simulink model "TST_Tra_GearInfo"  (R2016b)
settings: Solver=FixedStepDiscrete  StartTime=0.0  StopTime=simTime  FixedStep=sampleTime  RelTol=1e-3
values from neighbouring files (symbols this model uses):
  testCase = 1    [initTST_Tra_GearInfo_001.m]
libraries: simulink x11, UnitTest_Lib x9
settings Model: Creator=zhengjinyan  LastModifiedBy=zhengjinyan
settings DebuggingCC: SignalRangeChecking=error

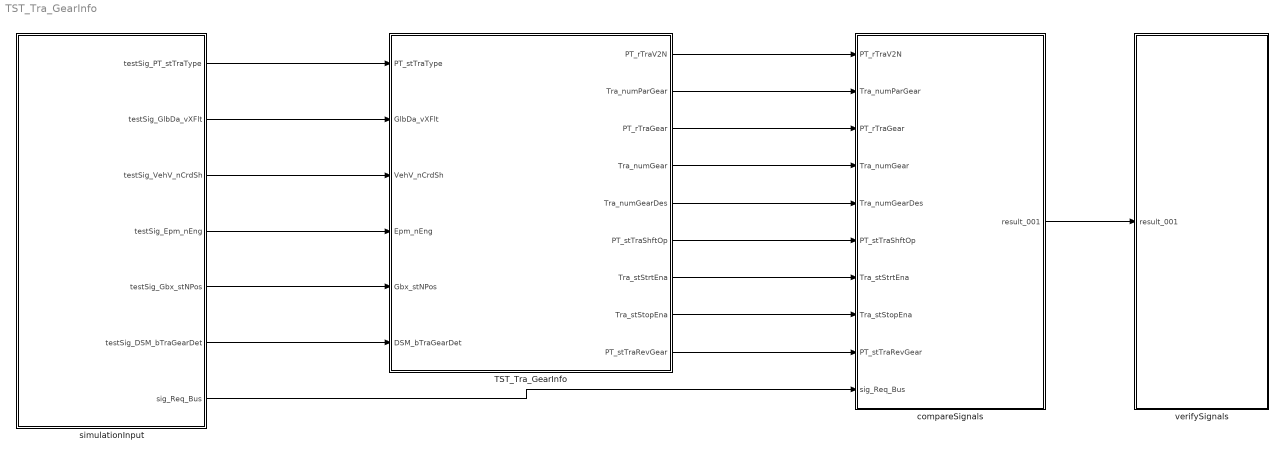
== system TST_Tra_GearInfo ==
  TST_Tra_GearInfo : Subsystem
  compareSignals : Subsystem
  simulationInput : Subsystem
  verifySignals : Subsystem
  wires:
  simulationInput/1(testSig_PT_stTraType) -> TST_Tra_GearInfo/1(PT_stTraType)
  simulationInput/2(testSig_GlbDa_vXFlt) -> TST_Tra_GearInfo/2(GlbDa_vXFlt)
  simulationInput/3(testSig_VehV_nCrdSh) -> TST_Tra_GearInfo/3(VehV_nCrdSh)
  simulationInput/4(testSig_Epm_nEng) -> TST_Tra_GearInfo/4(Epm_nEng)
  simulationInput/5(testSig_Gbx_stNPos) -> TST_Tra_GearInfo/5(Gbx_stNPos)
  simulationInput/6(testSig_DSM_bTraGearDet) -> TST_Tra_GearInfo/6(DSM_bTraGearDet)
  TST_Tra_GearInfo/1(PT_rTraV2N) -> compareSignals/1(PT_rTraV2N)
  TST_Tra_GearInfo/2(Tra_numParGear) -> compareSignals/2(Tra_numParGear)
  TST_Tra_GearInfo/3(PT_rTraGear) -> compareSignals/3(PT_rTraGear)
  TST_Tra_GearInfo/4(Tra_numGear) -> compareSignals/4(Tra_numGear)
  TST_Tra_GearInfo/5(Tra_numGearDes) -> compareSignals/5(Tra_numGearDes)
  TST_Tra_GearInfo/6(PT_stTraShftOp) -> compareSignals/6(PT_stTraShftOp)
  TST_Tra_GearInfo/7(Tra_stStrtEna) -> compareSignals/7(Tra_stStrtEna)
  TST_Tra_GearInfo/8(Tra_stStopEna) -> compareSignals/8(Tra_stStopEna)
  TST_Tra_GearInfo/9(PT_stTraRevGear) -> compareSignals/9(PT_stTraRevGear)
  simulationInput/7(sig_Req_Bus) -> compareSignals/10(sig_Req_Bus)
  compareSignals/1(result_001) -> verifySignals/1(result_001)

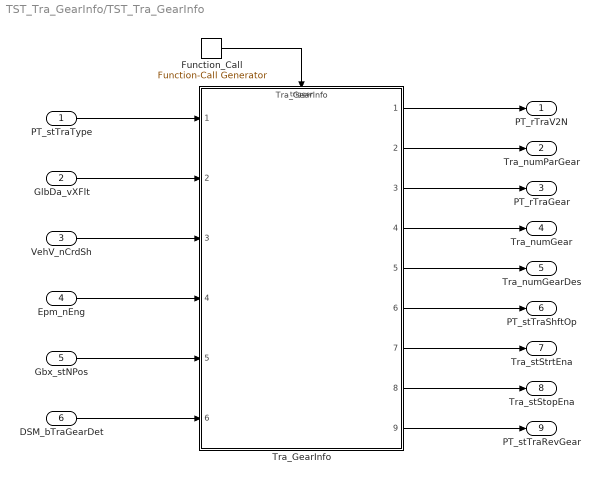
== system TST_Tra_GearInfo/TST_Tra_GearInfo ==
  PT_stTraType : Inport
  GlbDa_vXFlt : Inport  Port=2
  VehV_nCrdSh : Inport  Port=3
  Epm_nEng : Inport  Port=4
  Gbx_stNPos : Inport  Port=5
  DSM_bTraGearDet : Inport  Port=6
  Function_Call : simulink/Ports & Subsystems/Function-Call Generator  sample_time=sampleTime  numberOfIterations=1
  Tra_GearInfo : ModelReference  ModelNameDialog=Tra_GearInfo  SimulationMode=Normal  ModelReferenceVersion=1.62  TriggerPortName=function  TriggerPortTriggerType=function-call  TriggerPortStatesWhenEnabling=held
  PT_rTraV2N : Outport
  Tra_numParGear : Outport  Port=2
  PT_rTraGear : Outport  Port=3
  Tra_numGear : Outport  Port=4
  Tra_numGearDes : Outport  Port=5
  PT_stTraShftOp : Outport  Port=6
  Tra_stStrtEna : Outport  Port=7
  Tra_stStopEna : Outport  Port=8
  PT_stTraRevGear : Outport  Port=9
  wires:
  Function_Call/1 -> Tra_GearInfo/Trigger
  PT_stTraType/1 -> Tra_GearInfo/1
  GlbDa_vXFlt/1 -> Tra_GearInfo/2
  VehV_nCrdSh/1 -> Tra_GearInfo/3
  Epm_nEng/1 -> Tra_GearInfo/4
  Gbx_stNPos/1 -> Tra_GearInfo/5
  DSM_bTraGearDet/1 -> Tra_GearInfo/6
  Tra_GearInfo/1 -> PT_rTraV2N/1
  Tra_GearInfo/2 -> Tra_numParGear/1
  Tra_GearInfo/3 -> PT_rTraGear/1
  Tra_GearInfo/4 -> Tra_numGear/1
  Tra_GearInfo/5 -> Tra_numGearDes/1
  Tra_GearInfo/6 -> PT_stTraShftOp/1
  Tra_GearInfo/7 -> Tra_stStrtEna/1
  Tra_GearInfo/8 -> Tra_stStopEna/1
  Tra_GearInfo/9 -> PT_stTraRevGear/1

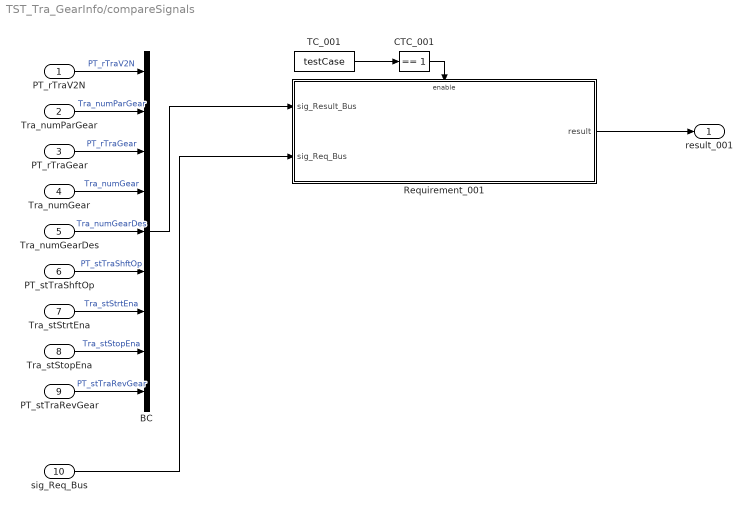
== system TST_Tra_GearInfo/compareSignals ==
  PT_rTraV2N : Inport
  Tra_numParGear : Inport  Port=2
  PT_rTraGear : Inport  Port=3
  Tra_numGear : Inport  Port=4
  Tra_numGearDes : Inport  Port=5
  PT_stTraShftOp : Inport  Port=6
  Tra_stStrtEna : Inport  Port=7
  Tra_stStopEna : Inport  Port=8
  PT_stTraRevGear : Inport  Port=9
  sig_Req_Bus : Inport  Port=10
  BC : BusCreator  Inputs=9
  CTC_001 : simulink/Logic and Bit Operations/Compare To Constant  relop===  const=1  OutDataTypeStr=boolean
  Requirement_001 : Subsystem
  TC_001 : Constant  Value=testCase
  result_001 : Outport
  wires:
  PT_rTraV2N/1 -> BC/1  "PT_rTraV2N"
  Tra_numParGear/1 -> BC/2  "Tra_numParGear"
  PT_rTraGear/1 -> BC/3  "PT_rTraGear"
  Tra_numGear/1 -> BC/4  "Tra_numGear"
  Tra_numGearDes/1 -> BC/5  "Tra_numGearDes"
  PT_stTraShftOp/1 -> BC/6  "PT_stTraShftOp"
  Tra_stStrtEna/1 -> BC/7  "Tra_stStrtEna"
  Tra_stStopEna/1 -> BC/8  "Tra_stStopEna"
  PT_stTraRevGear/1 -> BC/9  "PT_stTraRevGear"
  TC_001/1 -> CTC_001/1
  CTC_001/1 -> Requirement_001/Enable
  sig_Req_Bus/1 -> Requirement_001/2(sig_Req_Bus)
  BC/1 -> Requirement_001/1(sig_Result_Bus)
  Requirement_001/1(result) -> result_001/1

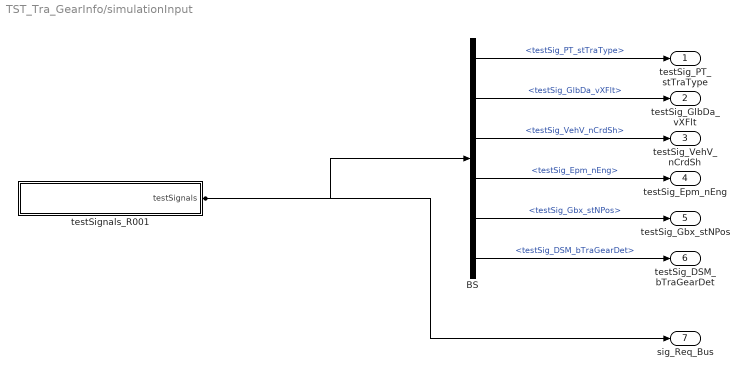
== system TST_Tra_GearInfo/simulationInput ==
  BS : BusSelector  OutputSignals=testSig_PT_stTraType,testSig_GlbDa_vXFlt,testSig_VehV_nCrdSh,testSig_Epm_nEng,testSig_Gbx_stNPos,testSig_DSM_bTraGearDet
  testSignals_R001 : Subsystem
  testSig_PT_stTraType : Outport
  testSig_GlbDa_vXFlt : Outport  Port=2
  testSig_VehV_nCrdSh : Outport  Port=3
  testSig_Epm_nEng : Outport  Port=4
  testSig_Gbx_stNPos : Outport  Port=5
  testSig_DSM_bTraGearDet : Outport  Port=6
  sig_Req_Bus : Outport  Port=7
  wires:
  BS/1 -> testSig_PT_stTraType/1  "<testSig_PT_stTraType>"
  BS/2 -> testSig_GlbDa_vXFlt/1  "<testSig_GlbDa_vXFlt>"
  BS/3 -> testSig_VehV_nCrdSh/1  "<testSig_VehV_nCrdSh>"
  BS/4 -> testSig_Epm_nEng/1  "<testSig_Epm_nEng>"
  BS/5 -> testSig_Gbx_stNPos/1  "<testSig_Gbx_stNPos>"
  BS/6 -> testSig_DSM_bTraGearDet/1  "<testSig_DSM_bTraGearDet>"
  testSignals_R001/1(testSignals) -> BS/1, sig_Req_Bus/1

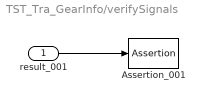
== system TST_Tra_GearInfo/verifySignals ==
  result_001 : Inport
  Assertion_001 : Assertion  Enabled=off
  wires:
  result_001/1 -> Assertion_001/1

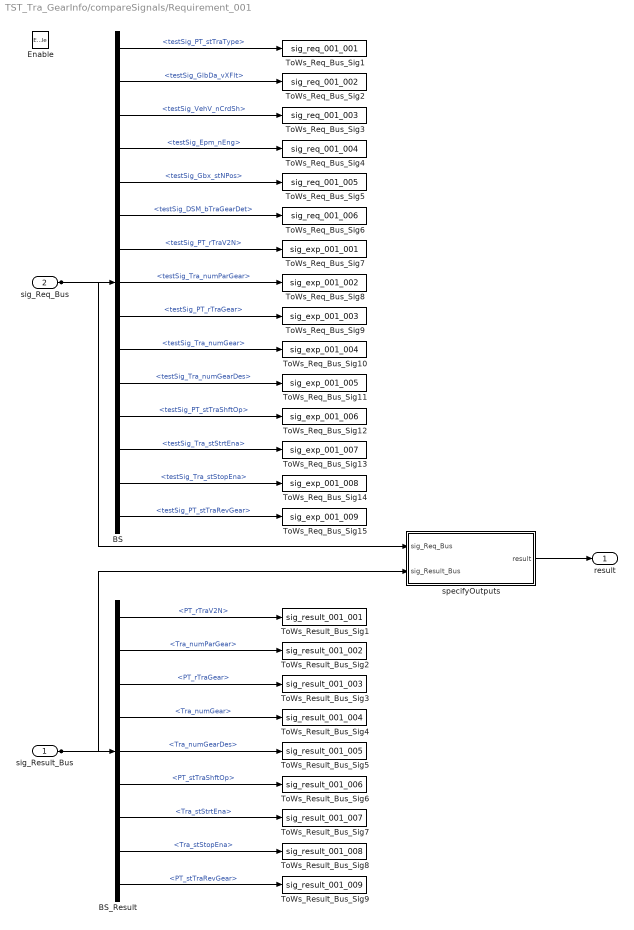
== system TST_Tra_GearInfo/compareSignals/Requirement_001 ==
  sig_Result_Bus : Inport
  sig_Req_Bus : Inport  Port=2
  Enable : EnablePort
  BS : BusSelector  OutputSignals=testSig_PT_stTraType,testSig_GlbDa_vXFlt,testSig_VehV_nCrdSh,testSig_Epm_nEng,testSig_Gbx_stNPos,testSig_DSM_bTraGearDet,testSig_PT_rTraV2N,testSig_Tra_numParGear,testSig_PT_rTraGear,testSig_Tra_numGear,testSig_Tra_numGearDes,testSig_PT_stTraShftOp,testSig_Tra_stStrtEna,testSig_Tra_stStopEna,testSig_PT_stTraRevGear
  BS_Result : BusSelector  OutputSignals=PT_rTraV2N,Tra_numParGear,PT_rTraGear,Tra_numGear,Tra_numGearDes,PT_stTraShftOp,Tra_stStrtEna,Tra_stStopEna,PT_stTraRevGear
  ToWs_Req_Bus_Sig1 : ToWorkspace  VariableName=sig_req_001_001  SaveFormat=Structure With Time
  ToWs_Req_Bus_Sig10 : ToWorkspace  VariableName=sig_exp_001_004  SaveFormat=Structure With Time
  ToWs_Req_Bus_Sig11 : ToWorkspace  VariableName=sig_exp_001_005  SaveFormat=Structure With Time
  ToWs_Req_Bus_Sig12 : ToWorkspace  VariableName=sig_exp_001_006  SaveFormat=Structure With Time
  ToWs_Req_Bus_Sig13 : ToWorkspace  VariableName=sig_exp_001_007  SaveFormat=Structure With Time
  ToWs_Req_Bus_Sig14 : ToWorkspace  VariableName=sig_exp_001_008  SaveFormat=Structure With Time
  ToWs_Req_Bus_Sig15 : ToWorkspace  VariableName=sig_exp_001_009  SaveFormat=Structure With Time
  ToWs_Req_Bus_Sig2 : ToWorkspace  VariableName=sig_req_001_002  SaveFormat=Structure With Time
  ToWs_Req_Bus_Sig3 : ToWorkspace  VariableName=sig_req_001_003  SaveFormat=Structure With Time
  ToWs_Req_Bus_Sig4 : ToWorkspace  VariableName=sig_req_001_004  SaveFormat=Structure With Time
  ToWs_Req_Bus_Sig5 : ToWorkspace  VariableName=sig_req_001_005  SaveFormat=Structure With Time
  ToWs_Req_Bus_Sig6 : ToWorkspace  VariableName=sig_req_001_006  SaveFormat=Structure With Time
  ToWs_Req_Bus_Sig7 : ToWorkspace  VariableName=sig_exp_001_001  SaveFormat=Structure With Time
  ToWs_Req_Bus_Sig8 : ToWorkspace  VariableName=sig_exp_001_002  SaveFormat=Structure With Time
  ToWs_Req_Bus_Sig9 : ToWorkspace  VariableName=sig_exp_001_003  SaveFormat=Structure With Time
  ToWs_Result_Bus_Sig1 : ToWorkspace  VariableName=sig_result_001_001  SaveFormat=Structure With Time
  ToWs_Result_Bus_Sig2 : ToWorkspace  VariableName=sig_result_001_002  SaveFormat=Structure With Time
  ToWs_Result_Bus_Sig3 : ToWorkspace  VariableName=sig_result_001_003  SaveFormat=Structure With Time
  ToWs_Result_Bus_Sig4 : ToWorkspace  VariableName=sig_result_001_004  SaveFormat=Structure With Time
  ToWs_Result_Bus_Sig5 : ToWorkspace  VariableName=sig_result_001_005  SaveFormat=Structure With Time
  ToWs_Result_Bus_Sig6 : ToWorkspace  VariableName=sig_result_001_006  SaveFormat=Structure With Time
  ToWs_Result_Bus_Sig7 : ToWorkspace  VariableName=sig_result_001_007  SaveFormat=Structure With Time
  ToWs_Result_Bus_Sig8 : ToWorkspace  VariableName=sig_result_001_008  SaveFormat=Structure With Time
  ToWs_Result_Bus_Sig9 : ToWorkspace  VariableName=sig_result_001_009  SaveFormat=Structure With Time
  specifyOutputs : Subsystem
  result : Outport
  wires:
  sig_Req_Bus/1 -> BS/1, specifyOutputs/1(sig_Req_Bus)
  BS/1 -> ToWs_Req_Bus_Sig1/1  "<testSig_PT_stTraType>"
  BS/2 -> ToWs_Req_Bus_Sig2/1  "<testSig_GlbDa_vXFlt>"
  BS/3 -> ToWs_Req_Bus_Sig3/1  "<testSig_VehV_nCrdSh>"
  BS/4 -> ToWs_Req_Bus_Sig4/1  "<testSig_Epm_nEng>"
  BS/5 -> ToWs_Req_Bus_Sig5/1  "<testSig_Gbx_stNPos>"
  BS/6 -> ToWs_Req_Bus_Sig6/1  "<testSig_DSM_bTraGearDet>"
  BS/7 -> ToWs_Req_Bus_Sig7/1  "<testSig_PT_rTraV2N>"
  BS/8 -> ToWs_Req_Bus_Sig8/1  "<testSig_Tra_numParGear>"
  BS/9 -> ToWs_Req_Bus_Sig9/1  "<testSig_PT_rTraGear>"
  BS/10 -> ToWs_Req_Bus_Sig10/1  "<testSig_Tra_numGear>"
  BS/11 -> ToWs_Req_Bus_Sig11/1  "<testSig_Tra_numGearDes>"
  BS/12 -> ToWs_Req_Bus_Sig12/1  "<testSig_PT_stTraShftOp>"
  BS/13 -> ToWs_Req_Bus_Sig13/1  "<testSig_Tra_stStrtEna>"
  BS/14 -> ToWs_Req_Bus_Sig14/1  "<testSig_Tra_stStopEna>"
  BS/15 -> ToWs_Req_Bus_Sig15/1  "<testSig_PT_stTraRevGear>"
  sig_Result_Bus/1 -> BS_Result/1, specifyOutputs/2(sig_Result_Bus)
  BS_Result/1 -> ToWs_Result_Bus_Sig1/1  "<PT_rTraV2N>"
  BS_Result/2 -> ToWs_Result_Bus_Sig2/1  "<Tra_numParGear>"
  BS_Result/3 -> ToWs_Result_Bus_Sig3/1  "<PT_rTraGear>"
  BS_Result/4 -> ToWs_Result_Bus_Sig4/1  "<Tra_numGear>"
  BS_Result/5 -> ToWs_Result_Bus_Sig5/1  "<Tra_numGearDes>"
  BS_Result/6 -> ToWs_Result_Bus_Sig6/1  "<PT_stTraShftOp>"
  BS_Result/7 -> ToWs_Result_Bus_Sig7/1  "<Tra_stStrtEna>"
  BS_Result/8 -> ToWs_Result_Bus_Sig8/1  "<Tra_stStopEna>"
  BS_Result/9 -> ToWs_Result_Bus_Sig9/1  "<PT_stTraRevGear>"
  specifyOutputs/1(result) -> result/1

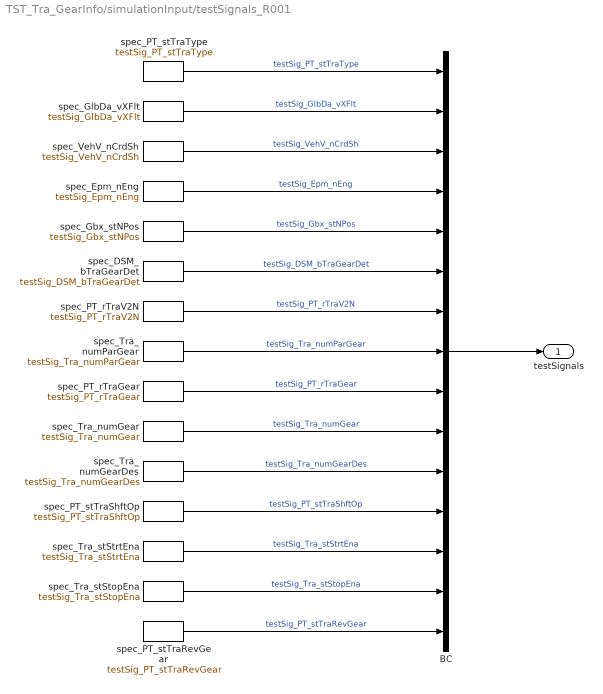
== system TST_Tra_GearInfo/simulationInput/testSignals_R001 ==
  BC : BusCreator  Inputs=15
  spec_DSM_bTraGearDet : FromWorkspace  VariableName=testSig_DSM_bTraGearDet  Interpolate=off  OutputAfterFinalValue=Holding final value
  spec_Epm_nEng : FromWorkspace  VariableName=testSig_Epm_nEng  Interpolate=off  OutputAfterFinalValue=Holding final value
  spec_Gbx_stNPos : FromWorkspace  VariableName=testSig_Gbx_stNPos  Interpolate=off  OutputAfterFinalValue=Holding final value
  spec_GlbDa_vXFlt : FromWorkspace  VariableName=testSig_GlbDa_vXFlt  Interpolate=off  OutputAfterFinalValue=Holding final value
  spec_PT_rTraGear : FromWorkspace  VariableName=testSig_PT_rTraGear  Interpolate=off  OutputAfterFinalValue=Holding final value
  spec_PT_rTraV2N : FromWorkspace  VariableName=testSig_PT_rTraV2N  Interpolate=off  OutputAfterFinalValue=Holding final value
  spec_PT_stTraRevGear : FromWorkspace  VariableName=testSig_PT_stTraRevGear  Interpolate=off  OutputAfterFinalValue=Holding final value
  spec_PT_stTraShftOp : FromWorkspace  VariableName=testSig_PT_stTraShftOp  Interpolate=off  OutputAfterFinalValue=Holding final value
  spec_PT_stTraType : FromWorkspace  VariableName=testSig_PT_stTraType  Interpolate=off  OutputAfterFinalValue=Holding final value
  spec_Tra_numGear : FromWorkspace  VariableName=testSig_Tra_numGear  Interpolate=off  OutputAfterFinalValue=Holding final value
  spec_Tra_numGearDes : FromWorkspace  VariableName=testSig_Tra_numGearDes  Interpolate=off  OutputAfterFinalValue=Holding final value
  spec_Tra_numParGear : FromWorkspace  VariableName=testSig_Tra_numParGear  Interpolate=off  OutputAfterFinalValue=Holding final value
  spec_Tra_stStopEna : FromWorkspace  VariableName=testSig_Tra_stStopEna  Interpolate=off  OutputAfterFinalValue=Holding final value
  spec_Tra_stStrtEna : FromWorkspace  VariableName=testSig_Tra_stStrtEna  Interpolate=off  OutputAfterFinalValue=Holding final value
  spec_VehV_nCrdSh : FromWorkspace  VariableName=testSig_VehV_nCrdSh  Interpolate=off  OutputAfterFinalValue=Holding final value
  testSignals : Outport
  wires:
  BC/1 -> testSignals/1
  spec_PT_stTraType/1 -> BC/1  "testSig_PT_stTraType"
  spec_GlbDa_vXFlt/1 -> BC/2  "testSig_GlbDa_vXFlt"
  spec_VehV_nCrdSh/1 -> BC/3  "testSig_VehV_nCrdSh"
  spec_Epm_nEng/1 -> BC/4  "testSig_Epm_nEng"
  spec_Gbx_stNPos/1 -> BC/5  "testSig_Gbx_stNPos"
  spec_DSM_bTraGearDet/1 -> BC/6  "testSig_DSM_bTraGearDet"
  spec_PT_rTraV2N/1 -> BC/7  "testSig_PT_rTraV2N"
  spec_Tra_numParGear/1 -> BC/8  "testSig_Tra_numParGear"
  spec_PT_rTraGear/1 -> BC/9  "testSig_PT_rTraGear"
  spec_Tra_numGear/1 -> BC/10  "testSig_Tra_numGear"
  spec_Tra_numGearDes/1 -> BC/11  "testSig_Tra_numGearDes"
  spec_PT_stTraShftOp/1 -> BC/12  "testSig_PT_stTraShftOp"
  spec_Tra_stStrtEna/1 -> BC/13  "testSig_Tra_stStrtEna"
  spec_Tra_stStopEna/1 -> BC/14  "testSig_Tra_stStopEna"
  spec_PT_stTraRevGear/1 -> BC/15  "testSig_PT_stTraRevGear"

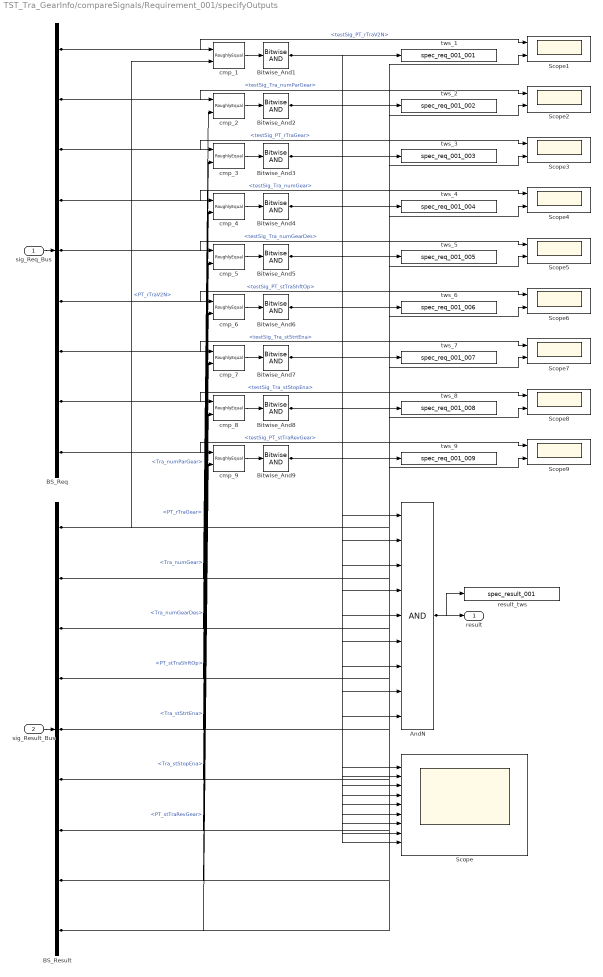
== system TST_Tra_GearInfo/compareSignals/Requirement_001/specifyOutputs ==
  sig_Req_Bus : Inport
  sig_Result_Bus : Inport  Port=2
  AndN : Logic  Inputs=9
  BS_Req : BusSelector  OutputSignals=testSig_PT_rTraV2N,testSig_Tra_numParGear,testSig_PT_rTraGear,testSig_Tra_numGear,testSig_Tra_numGearDes,testSig_PT_stTraShftOp,testSig_Tra_stStrtEna,testSig_Tra_stStopEna,testSig_PT_stTraRevGear
  BS_Result : BusSelector  OutputSignals=PT_rTraV2N,Tra_numParGear,PT_rTraGear,Tra_numGear,Tra_numGearDes,PT_stTraShftOp,Tra_stStrtEna,Tra_stStopEna,PT_stTraRevGear
  Bitwise_And{1..9} (9 alike) : simulink/Logic and Bit Operations/Bitwise Operator  logicop=AND  UseBitMask=off  BitMask=bin2dec('11011001')  BitMaskRealWorld=Stored Integer
  Scope : Scope  NumInputPorts=9
  Scope{1..9} (9 alike) : Scope  NumInputPorts=2
  cmp_{1..9} (9 alike) : UnitTest_Lib/RoughlyEqual  slope=0.1
  result_tws : ToWorkspace  VariableName=spec_result_001
  tws_1 : ToWorkspace  VariableName=spec_req_001_001
  tws_2 : ToWorkspace  VariableName=spec_req_001_002
  tws_3 : ToWorkspace  VariableName=spec_req_001_003
  tws_4 : ToWorkspace  VariableName=spec_req_001_004
  tws_5 : ToWorkspace  VariableName=spec_req_001_005
  tws_6 : ToWorkspace  VariableName=spec_req_001_006
  tws_7 : ToWorkspace  VariableName=spec_req_001_007
  tws_8 : ToWorkspace  VariableName=spec_req_001_008
  tws_9 : ToWorkspace  VariableName=spec_req_001_009
  result : Outport
  wires:
  sig_Req_Bus/1 -> BS_Req/1
  sig_Result_Bus/1 -> BS_Result/1
  AndN/1 -> result/1, result_tws/1
  BS_Req/1 -> cmp_1/1, Scope1/1  "<testSig_PT_rTraV2N>"
  BS_Result/1 -> cmp_1/2, Scope1/2  "<PT_rTraV2N>"
  cmp_1/1 -> Bitwise_And1/1
  Bitwise_And1/1 -> tws_1/1, AndN/1, Scope/1
  BS_Req/2 -> cmp_2/1, Scope2/1  "<testSig_Tra_numParGear>"
  BS_Result/2 -> cmp_2/2, Scope2/2  "<Tra_numParGear>"
  cmp_2/1 -> Bitwise_And2/1
  Bitwise_And2/1 -> tws_2/1, AndN/2, Scope/2
  BS_Req/3 -> cmp_3/1, Scope3/1  "<testSig_PT_rTraGear>"
  BS_Result/3 -> cmp_3/2, Scope3/2  "<PT_rTraGear>"
  cmp_3/1 -> Bitwise_And3/1
  Bitwise_And3/1 -> tws_3/1, AndN/3, Scope/3
  BS_Req/4 -> cmp_4/1, Scope4/1  "<testSig_Tra_numGear>"
  BS_Result/4 -> cmp_4/2, Scope4/2  "<Tra_numGear>"
  cmp_4/1 -> Bitwise_And4/1
  Bitwise_And4/1 -> tws_4/1, AndN/4, Scope/4
  BS_Req/5 -> cmp_5/1, Scope5/1  "<testSig_Tra_numGearDes>"
  BS_Result/5 -> cmp_5/2, Scope5/2  "<Tra_numGearDes>"
  cmp_5/1 -> Bitwise_And5/1
  Bitwise_And5/1 -> tws_5/1, AndN/5, Scope/5
  BS_Req/6 -> cmp_6/1, Scope6/1  "<testSig_PT_stTraShftOp>"
  BS_Result/6 -> cmp_6/2, Scope6/2  "<PT_stTraShftOp>"
  cmp_6/1 -> Bitwise_And6/1
  Bitwise_And6/1 -> tws_6/1, AndN/6, Scope/6
  BS_Req/7 -> cmp_7/1, Scope7/1  "<testSig_Tra_stStrtEna>"
  BS_Result/7 -> cmp_7/2, Scope7/2  "<Tra_stStrtEna>"
  cmp_7/1 -> Bitwise_And7/1
  Bitwise_And7/1 -> tws_7/1, AndN/7, Scope/7
  BS_Req/8 -> cmp_8/1, Scope8/1  "<testSig_Tra_stStopEna>"
  BS_Result/8 -> cmp_8/2, Scope8/2  "<Tra_stStopEna>"
  cmp_8/1 -> Bitwise_And8/1
  Bitwise_And8/1 -> tws_8/1, AndN/8, Scope/8
  BS_Req/9 -> cmp_9/1, Scope9/1  "<testSig_PT_stTraRevGear>"
  BS_Result/9 -> cmp_9/2, Scope9/2  "<PT_stTraRevGear>"
  cmp_9/1 -> Bitwise_And9/1
  Bitwise_And9/1 -> tws_9/1, AndN/9, Scope/9
